simulink model "s_ks_estudio_final"  (R2022b)
settings: Solver=VariableStepAuto  StartTime=0.0  StopTime=200  RelTol=1e-3
libraries: fuzblock x8, simulink x1
settings Model: Creator=sophy  LastModifiedBy=sophy

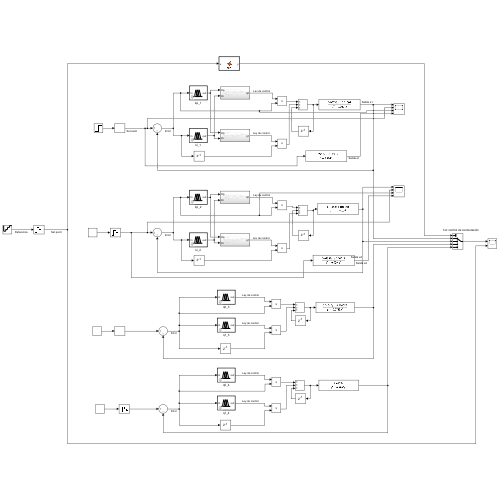
[thumbnail: Simulink's stored preview of the top-level diagram]
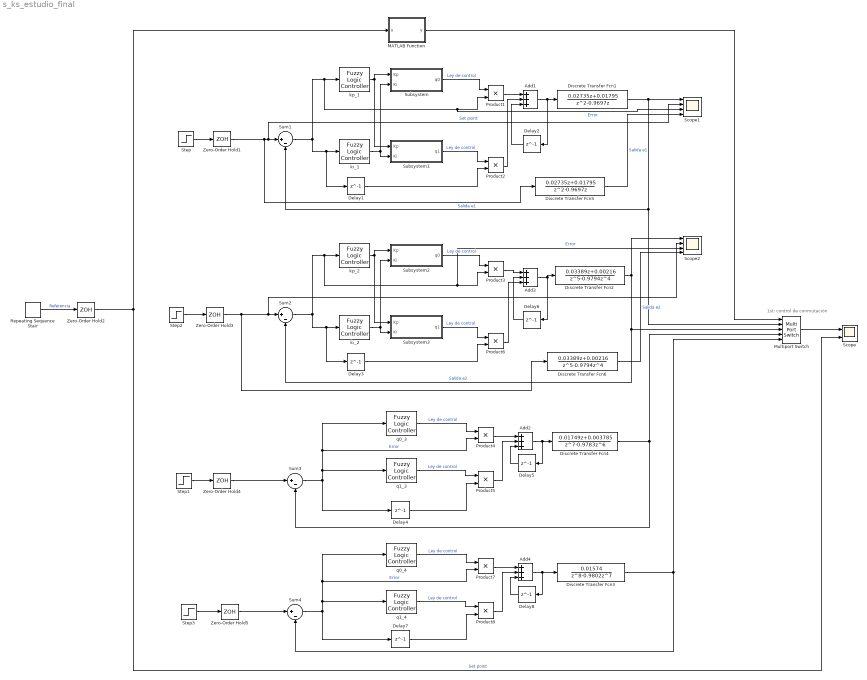
== system s_ks_estudio_final ==
  note: 1st: control de conmutación
  Add{1..4} (4 alike) : Sum  Inputs=+++
  Delay{1..8} (8 alike) : Delay  DelayLength=1
  Discrete Transfer Fcn1 : DiscreteTransferFcn  Numerator=[0.02735 0.01795]  Denominator=[1 -0.9697 0]
  Discrete Transfer Fcn2 : DiscreteTransferFcn  Numerator=[0.03389 0.00216]  Denominator=[1 -0.9794 0 0 0 0]
  Discrete Transfer Fcn3 : DiscreteTransferFcn  Numerator=[0.01574]  Denominator=[1 -0.9802 0 0 0 0 0 0 0]
  Discrete Transfer Fcn4 : DiscreteTransferFcn  Numerator=[0.01749 0.003785]  Denominator=[1 -0.9783 0 0 0 0 0 0]
  Discrete Transfer Fcn5 : DiscreteTransferFcn  Numerator=[0.02735 0.01795]  Denominator=[1 -0.9697 0]
  Discrete Transfer Fcn6 : DiscreteTransferFcn  Numerator=[0.03389 0.00216]  Denominator=[1 -0.9794 0 0 0 0]
  MATLAB Function : MATLAB Function  TreatAsAtomicUnit=on
  Multiport Switch : MultiPortSwitch  Inputs=4  SaturateOnIntegerOverflow=off  InputSameDT=off
  Product{1..8} (8 alike) : Product
  Repeating Sequence Stair : simulink/Sources/Repeating Sequence Stair  OutValues=[20 30 40 50].'  tsamp=50  OutMin=[]  OutMax=[]  OutDataTypeStr=double  OutputDataTypeScalingMode=double  OutDataType=fixdt(0,8)  ConRadixGroup=Best Precision: Vector-wise  OutScaling=2^-12
  Scope : Scope  NumInputPorts=2
  Scope1 : Scope  NumInputPorts=4
  Scope2 : Scope  NumInputPorts=4
  Step : Step  After=20  SampleTime=0
  Step1 : Step  After=10  SampleTime=0
  Step2 : Step  After=10  SampleTime=0
  Step3 : Step  After=10  SampleTime=0
  Subsystem : Subsystem
  Subsystem1 : Subsystem
  Subsystem2 : Subsystem
  Subsystem3 : Subsystem
  Sum{1..4} (4 alike) : Sum  Inputs=|+-
  Zero-Order Hold{1,3..5} (4 alike) : ZeroOrderHold
  Zero-Order Hold2 : ZeroOrderHold  SampleTime=0.2
  ki_1 : fuzblock/Fuzzy Logic  Controller  FIS=q1_e1  OutputSampleNumber=101  DataType=double  FuzzifiedInputs=off  RuleFiringStrengths=off  RuleOutputs=off  AggregatedOutputs=off  SimulateUsing=Interpreted execution  OutOfRangeInputValueMessage=warning  NoRuleFiredMessage=warning  EmptyOutputFuzzySetMessage=warning
  ki_2 : fuzblock/Fuzzy Logic  Controller  FIS=ki_e2  OutputSampleNumber=101  DataType=double  FuzzifiedInputs=off  RuleFiringStrengths=off  RuleOutputs=off  AggregatedOutputs=off  SimulateUsing=Interpreted execution  OutOfRangeInputValueMessage=warning  NoRuleFiredMessage=warning  EmptyOutputFuzzySetMessage=warning
  kp_1 : fuzblock/Fuzzy Logic  Controller  FIS=q0_e1  OutputSampleNumber=101  DataType=double  FuzzifiedInputs=off  RuleFiringStrengths=off  RuleOutputs=off  AggregatedOutputs=off  SimulateUsing=Interpreted execution  OutOfRangeInputValueMessage=warning  NoRuleFiredMessage=warning  EmptyOutputFuzzySetMessage=warning
  kp_2 : fuzblock/Fuzzy Logic  Controller  FIS=kp_e2  OutputSampleNumber=101  DataType=double  FuzzifiedInputs=off  RuleFiringStrengths=off  RuleOutputs=off  AggregatedOutputs=off  SimulateUsing=Interpreted execution  OutOfRangeInputValueMessage=warning  NoRuleFiredMessage=warning  EmptyOutputFuzzySetMessage=warning
  q0_3 : fuzblock/Fuzzy Logic  Controller  FIS=q0_PID  OutputSampleNumber=101  DataType=double  FuzzifiedInputs=off  RuleFiringStrengths=off  RuleOutputs=off  AggregatedOutputs=off  SimulateUsing=Interpreted execution  OutOfRangeInputValueMessage=warning  NoRuleFiredMessage=warning  EmptyOutputFuzzySetMessage=warning
  q0_4 : fuzblock/Fuzzy Logic  Controller  FIS=q0_PID  OutputSampleNumber=101  DataType=double  FuzzifiedInputs=off  RuleFiringStrengths=off  RuleOutputs=off  AggregatedOutputs=off  SimulateUsing=Interpreted execution  OutOfRangeInputValueMessage=warning  NoRuleFiredMessage=warning  EmptyOutputFuzzySetMessage=warning
  q1_3 : fuzblock/Fuzzy Logic  Controller  FIS=q1_PID  OutputSampleNumber=101  DataType=double  FuzzifiedInputs=off  RuleFiringStrengths=off  RuleOutputs=off  AggregatedOutputs=off  SimulateUsing=Interpreted execution  OutOfRangeInputValueMessage=warning  NoRuleFiredMessage=warning  EmptyOutputFuzzySetMessage=warning
  q1_4 : fuzblock/Fuzzy Logic  Controller  FIS=q1_PID  OutputSampleNumber=101  DataType=double  FuzzifiedInputs=off  RuleFiringStrengths=off  RuleOutputs=off  AggregatedOutputs=off  SimulateUsing=Interpreted execution  OutOfRangeInputValueMessage=warning  NoRuleFiredMessage=warning  EmptyOutputFuzzySetMessage=warning
  wires:
  Product2/1 -> Add1/2
  Sum1/1 -> kp_1/1, Scope1/3, Product1/2, Delay1/1, ki_1/1  "Error"
  Repeating Sequence Stair/1 -> Zero-Order Hold2/1  "Referencia"
  Add1/1 -> Delay2/1, Discrete Transfer Fcn1/1
  Delay7/1 -> Product8/2
  Discrete Transfer Fcn4/1 -> Multiport Switch/4, Sum3/2
  Add2/1 -> Discrete Transfer Fcn4/1, Delay5/1
  Sum4/1 -> q0_4/1, Product7/2, q1_4/1, Delay7/1  "Error"
  Product8/1 -> Add4/2
  Delay4/1 -> Product5/2
  q1_3/1 -> Product5/1  "Ley de control"
  q0_4/1 -> Product7/1  "Ley de control"
  q0_3/1 -> Product4/1  "Ley de control"
  Delay5/1 -> Add2/3
  Discrete Transfer Fcn1/1 -> Scope1/1, Sum1/2, Multiport Switch/2  "Salida e1"
  MATLAB Function/1(y) -> Multiport Switch/1
  Discrete Transfer Fcn3/1 -> Multiport Switch/5, Sum4/2
  Product4/1 -> Add2/1
  Delay8/1 -> Add4/3
  Product7/1 -> Add4/1
  Product1/1 -> Add1/1
  Product5/1 -> Add2/2
  q1_4/1 -> Product8/1  "Ley de control"
  Delay1/1 -> Product2/2
  Add4/1 -> Delay8/1, Discrete Transfer Fcn3/1
  Multiport Switch/1 -> Scope/1
  Sum3/1 -> q0_3/1, Product4/2, q1_3/1, Delay4/1  "Error"
  Zero-Order Hold2/1 -> MATLAB Function/1(u), Scope/2  "Set point"
  Step/1 -> Zero-Order Hold1/1
  kp_1/1 -> Subsystem1/1(Kp), Subsystem/1(Kp)
  ki_1/1 -> Subsystem1/2(Ki), Subsystem/2(Ki)
  Subsystem/1(q0) -> Product1/1  "Ley de control"
  Subsystem1/1(q1) -> Product2/1  "Ley de control"
  Product6/1 -> Add3/3
  Sum2/1 -> kp_2/1, Scope2/3, Product3/2, Delay3/1, ki_2/1  "Error"
  ki_2/1 -> Subsystem3/2(Ki), Subsystem2/2(Ki)
  Delay6/1 -> Add3/2
  Delay3/1 -> Product6/2
  Discrete Transfer Fcn2/1 -> Scope2/1, Sum2/2, Multiport Switch/3  "Salida e2"
  Add3/1 -> Discrete Transfer Fcn2/1, Delay6/1
  Zero-Order Hold3/1 -> Discrete Transfer Fcn6/1, Scope2/2, Sum2/1
  Product3/1 -> Add3/1
  Subsystem3/1(q1) -> Product6/1  "Ley de control"
  Subsystem2/1(q0) -> Product3/1  "Ley de control"
  kp_2/1 -> Subsystem3/1(Kp), Subsystem2/1(Kp)
  Delay2/1 -> Add1/3
  Zero-Order Hold1/1 -> Discrete Transfer Fcn5/1, Scope1/2, Sum1/1  "Set point"
  Discrete Transfer Fcn5/1 -> Scope1/4  "Salida e1"
  Step2/1 -> Zero-Order Hold3/1
  Step1/1 -> Zero-Order Hold4/1
  Step3/1 -> Zero-Order Hold5/1
  Zero-Order Hold5/1 -> Sum4/1
  Zero-Order Hold4/1 -> Sum3/1
  Discrete Transfer Fcn6/1 -> Scope2/4  "Salida e2"

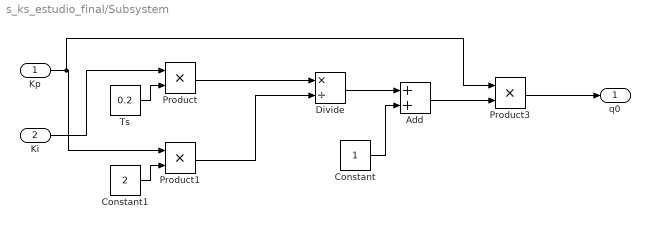
== system s_ks_estudio_final/Subsystem ==
  Kp : Inport
  Ki : Inport  Port=2
  Add : Sum
  Constant : Constant
  Constant1 : Constant  Value=2
  Divide : Product  Inputs=*/
  Product : Product
  Product1 : Product
  Product3 : Product
  Ts : Constant  Value=0.2
  q0 : Outport
  wires:
  Constant/1 -> Add/2
  Ki/1 -> Product/1
  Ts/1 -> Product/2
  Product/1 -> Divide/1
  Constant1/1 -> Product1/2
  Kp/1 -> Product3/1, Product1/1
  Product1/1 -> Divide/2
  Divide/1 -> Add/1
  Add/1 -> Product3/2
  Product3/1 -> q0/1

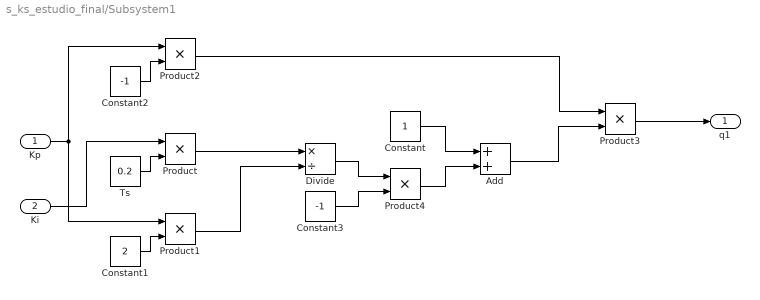
== system s_ks_estudio_final/Subsystem1 ==
  Kp : Inport
  Ki : Inport  Port=2
  Add : Sum
  Constant : Constant
  Constant1 : Constant  Value=2
  Constant2 : Constant  Value=-1
  Constant3 : Constant  Value=-1
  Divide : Product  Inputs=*/
  Product{,1..4} (5 alike) : Product
  Ts : Constant  Value=0.2
  q1 : Outport
  wires:
  Constant/1 -> Add/1
  Ki/1 -> Product/1
  Ts/1 -> Product/2
  Product/1 -> Divide/1
  Constant1/1 -> Product1/2
  Kp/1 -> Product1/1, Product2/1
  Product1/1 -> Divide/2
  Product3/1 -> q1/1
  Constant2/1 -> Product2/2
  Product2/1 -> Product3/1
  Add/1 -> Product3/2
  Constant3/1 -> Product4/2
  Divide/1 -> Product4/1
  Product4/1 -> Add/2

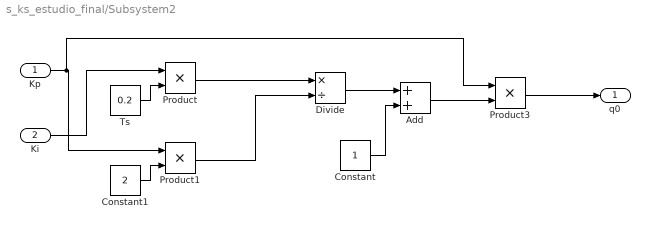
== system s_ks_estudio_final/Subsystem2 ==
  Kp : Inport
  Ki : Inport  Port=2
  Add : Sum
  Constant : Constant
  Constant1 : Constant  Value=2
  Divide : Product  Inputs=*/
  Product : Product
  Product1 : Product
  Product3 : Product
  Ts : Constant  Value=0.2
  q0 : Outport
  wires:
  Constant/1 -> Add/2
  Ki/1 -> Product/1
  Ts/1 -> Product/2
  Product/1 -> Divide/1
  Constant1/1 -> Product1/2
  Kp/1 -> Product3/1, Product1/1
  Product1/1 -> Divide/2
  Divide/1 -> Add/1
  Add/1 -> Product3/2
  Product3/1 -> q0/1

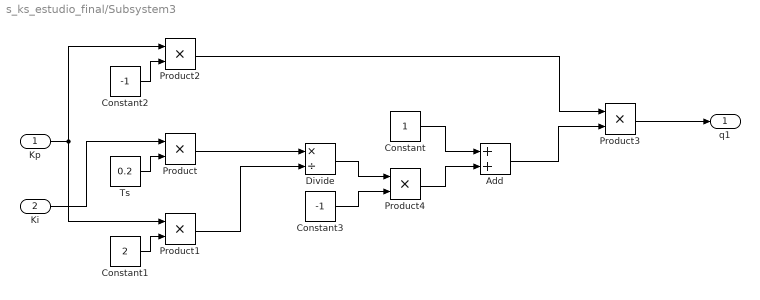
== system s_ks_estudio_final/Subsystem3 ==
  Kp : Inport
  Ki : Inport  Port=2
  Add : Sum
  Constant : Constant
  Constant1 : Constant  Value=2
  Constant2 : Constant  Value=-1
  Constant3 : Constant  Value=-1
  Divide : Product  Inputs=*/
  Product{,1..4} (5 alike) : Product
  Ts : Constant  Value=0.2
  q1 : Outport
  wires:
  Constant/1 -> Add/1
  Ki/1 -> Product/1
  Ts/1 -> Product/2
  Product/1 -> Divide/1
  Constant1/1 -> Product1/2
  Kp/1 -> Product1/1, Product2/1
  Product1/1 -> Divide/2
  Product3/1 -> q1/1
  Constant2/1 -> Product2/2
  Product2/1 -> Product3/1
  Add/1 -> Product3/2
  Constant3/1 -> Product4/2
  Divide/1 -> Product4/1
  Product4/1 -> Add/2

== matlab function s_ks_estudio_final/MATLAB Function ==
  data: u input; y output
function y = fcn(u)

if ((u>0)&&(u<=20)) % u = lo que entra = escalon
u = 1; % activar pin 1
end

if ((u>20)&&(u<=30))
u = 2; % activar pin 2
end 

if ((u>30)&&(u<=40))
u = 3; % activar pin 3
end 

if ((u>40)&&(u<=50))
u = 4; % activar pin 4
end 

y = u;
